simulink model "neurogrip_c0_closed_loop"  (R2026a)
settings: Solver=FixedStepDiscrete  StopTime=0.4  FixedStep=0.02
model workspace (MAT data in the model file):
  c0Mpc = mpc
  c0Mpc.Ts = 0.02
  c0Mpc.PredictionHorizon = 30
  c0Mpc.ControlHorizon = 30
  c0Mpc.Model.Plant = ss
  c0Mpc.Model.Plant.InputName_ = ["steering_angle_rad"; "d_kappa_rad_s"]
  c0Mpc.Model.Plant.InputGroup_.Manipulated = 1
  c0Mpc.Model.Plant.InputGroup_.Measured = 2
  c0Mpc.Model.Plant.OutputName_ = ["e_y_m"; "e_psi_rad"; "v_y_mps"; "yaw_rate_rps"]
  c0Mpc.Model.Plant.OutputGroup_.Measured = [1 2 3 4]
  c0Mpc.Model.Plant.IOSize_ = [4 2]
  c0Mpc.Model.Plant.Data_ = ltipack.ssdata
  c0Mpc.Model.Plant.Data_.a = [1  0.09  0.02  0; 0  1  0  0.02; 0  0  0.463654239616  -0.0414393740331; 0  0  0  0.457235651577]
  c0Mpc.Model.Plant.Data_.c = [1  0  0  0; 0  1  0  0; 0  0  1  0; 0  0  0  1]
  c0Mpc.Model.Plant.Data_.dx0 = [0; 0; 0; 0]
  c0Mpc.Model.Plant.Data_.x0 = [0; 0; 0; 0]
  c0Mpc.Model.Plant.Data_.b = [0  0; 0  -0.02; 1.14394485122  0; 1.59636573066  0]
  c0Mpc.Model.Plant.Data_.d = [0  0; 0  0; 0  0; 0  0]
  c0Mpc.Model.Plant.Data_.u0 = [0; 0]
  c0Mpc.Model.Plant.Data_.y0 = [0; 0; 0; 0]
  c0Mpc.Model.Plant.Data_.Delay.Input = [0; 0]
  c0Mpc.Model.Plant.Data_.Delay.Output = [0; 0; 0; 0]
  c0Mpc.Model.Plant.Data_.Delay.Internal = []
  c0Mpc.Model.Plant.Data_.Ts = 0.02
  c0Mpc.Model.Disturbance = []
  c0Mpc.Model.Noise = []
  c0Mpc.Model.Nominal.X = [0; 0; 0; 0]
  c0Mpc.Model.Nominal.DX = [0; 0; 0; 0]
  c0Mpc.Model.Nominal.U = [0; 0]
  c0Mpc.Model.Nominal.Y = [0; 0; 0; 0]
  c0Mpc.ManipulatedVariables.Min = -0.37
  c0Mpc.ManipulatedVariables.Max = 0.37
  c0Mpc.ManipulatedVariables.MinECR = 0
  c0Mpc.ManipulatedVariables.MaxECR = 0
  c0Mpc.ManipulatedVariables.RateMin = -0.05
  c0Mpc.ManipulatedVariables.RateMax = 0.05
  c0Mpc.ManipulatedVariables.RateMinECR = 0
  c0Mpc.ManipulatedVariables.RateMaxECR = 0
  c0Mpc.ManipulatedVariables.Target = 'nominal'
  c0Mpc.ManipulatedVariables.Name = 'steering_angle_rad'
  c0Mpc.ManipulatedVariables.Units = ''
  c0Mpc.ManipulatedVariables.ScaleFactor = 1
  c0Mpc.ManipulatedVariables.Type = 'continuous'
  c0Mpc.OutputVariables(1).Min = -1.5
  c0Mpc.OutputVariables(1).Max = 1.5
  c0Mpc.OutputVariables(1).MinECR = 1
  c0Mpc.OutputVariables(1).MaxECR = 1
  c0Mpc.OutputVariables(1).Name = 'e_y_m'
  c0Mpc.OutputVariables(1).Units = ''
  c0Mpc.OutputVariables(1).ScaleFactor = 1
  c0Mpc.OutputVariables(2).Min = -Inf
  c0Mpc.OutputVariables(2).Max = Inf
  c0Mpc.OutputVariables(2).MinECR = 1
  c0Mpc.OutputVariables(2).MaxECR = 1
  c0Mpc.OutputVariables(2).Name = 'e_psi_rad'
  c0Mpc.OutputVariables(2).Units = ''
  c0Mpc.OutputVariables(2).ScaleFactor = 1
  c0Mpc.OutputVariables(3).Min = -Inf
  c0Mpc.OutputVariables(3).Max = Inf
  c0Mpc.OutputVariables(3).MinECR = 1
  c0Mpc.OutputVariables(3).MaxECR = 1
  c0Mpc.OutputVariables(3).Name = 'v_y_mps'
  c0Mpc.OutputVariables(3).Units = ''
  c0Mpc.OutputVariables(3).ScaleFactor = 1
  c0Mpc.OutputVariables(4).Min = -Inf
  c0Mpc.OutputVariables(4).Max = Inf
  c0Mpc.OutputVariables(4).MinECR = 1
  c0Mpc.OutputVariables(4).MaxECR = 1
  c0Mpc.OutputVariables(4).Name = 'yaw_rate_rps'
  c0Mpc.OutputVariables(4).Units = ''
  c0Mpc.OutputVariables(4).ScaleFactor = 1
  c0Mpc.DisturbanceVariables.Name = 'd_kappa_rad_s'
  c0Mpc.DisturbanceVariables.Units = ''
  c0Mpc.DisturbanceVariables.ScaleFactor = 1
  c0Mpc.Weights.ManipulatedVariables = 20
  c0Mpc.Weights.ManipulatedVariablesRate = 5
  c0Mpc.Weights.OutputVariables = [40 60 5 10]
  c0Mpc.Weights.ECR = 100000
  c0Mpc.Optimizer.OptimizationType = 'QP'
  c0Mpc.Optimizer.Solver = 'active-set'
  c0Mpc.Optimizer.SolverOptions = mpc.solver.options.qp.ActiveSet
  c0Mpc.Optimizer.SolverOptions.SolverName = 'ActiveSet'
  c0Mpc.Optimizer.MinOutputECR = 0
  c0Mpc.Optimizer.UseSuboptimalSolution = 0
  c0Mpc.Optimizer.CustomSolver = 0
  c0Mpc.Optimizer.CustomSolverCodeGen = 0
  c0Mpc.History = [2026 10 3 11 47 54.765249]
  c0Mpc.MPCData = mpcdata
  c0Mpc.MPCData.IsDirty = 1
  c0Mpc.MPCData.Ts = 0.02
  c0Mpc.MPCData.p = 30
  c0Mpc.MPCData.m = 30
  c0Mpc.MPCData.UseActiveSetSolver = 1
  c0Mpc.MPCData.UseSuboptimalSolution = 0
  c0Mpc.MPCData.CustomSolver = 0
  c0Mpc.MPCData.CustomSolverCodeGen = 0
  c0Mpc.MPCData.IsCustomEstimation = 0
  c0Mpc.MPCData.Uscale = [1; 1]
  c0Mpc.MPCData.Yscale = [1; 1; 1; 1]
  c0Mpc.MPCData.mvindex = 1
  c0Mpc.MPCData.mdindex = 2
  c0Mpc.MPCData.myindex = [1; 2; 3; 4]
  c0Mpc.MPCData.ASOptions.MaxIterations = 120
  c0Mpc.MPCData.ASOptions.ConstraintTolerance = 1e-06
  c0Mpc.MPCData.ASOptions.UseWarmStart = 1
  c0Mpc.MPCData.IPOptions.MaxIterations = 50
  c0Mpc.MPCData.IPOptions.ConstraintTolerance = 1e-06
  c0Mpc.MPCData.IPOptions.OptimalityTolerance = 1e-06
  c0Mpc.MPCData.IPOptions.ComplementarityTolerance = 1e-08
  c0Mpc.MPCData.IPOptions.StepTolerance = 1e-08
  c0Mpc.MPCData.ADOptions.AbsoluteTolerance = 0.001
  c0Mpc.MPCData.ADOptions.RelativeTolerance = 0.001
  c0Mpc.MPCData.ADOptions.MaxIterations = 1000
  c0Mpc.MPCData.ADOptions.RelaxationParameter = 1.6
  c0Mpc.MPCData.ADOptions.PenaltyParameter = 0.1
  c0Mpc.MPCData.ADOptions.StepSize = 1e-06
  c0Mpc.MPCData.ADOptions.PrimalInfeasibilityTolerance = 0.0001
  c0Mpc.MPCData.ADOptions.DualInfeasibilityTolerance = 0.0001
  c0Mpc.MPCData.ADOptions.EnablePolish = 0
  c0Mpc.MPCData.ADOptions.PolishRegularization = 1e-06
  c0Mpc.MPCData.ADOptions.PolishTolerance = 1e-08
  c0Mpc.MPCData.ADOptions.PolishMaxIterations = 3
  c0Mpc.MPCData.MIQPOptions.MaxIterations = 1000
  c0Mpc.MPCData.MIQPOptions.ConstraintTolerance = 1e-06
  c0Mpc.MPCData.MIQPOptions.UseWarmStart = 0
  c0Mpc.MPCData.MIQPOptions.DiscreteConstraintTolerance = 1e-06
  c0Mpc.MPCData.MIQPOptions.RoundingAtRootNode = 1
  c0Mpc.MPCData.MIQPOptions.MaxPendingNodes = 1000
  c0Mpc.IsEmpty = 0
  c0Mpc.OldOVIntegrator = {[]; []; []; []}
  c0Mpc.Version = '26.1'
libraries: mpclib x1
settings Model: Creator=pavel  LastModifiedBy=pavel

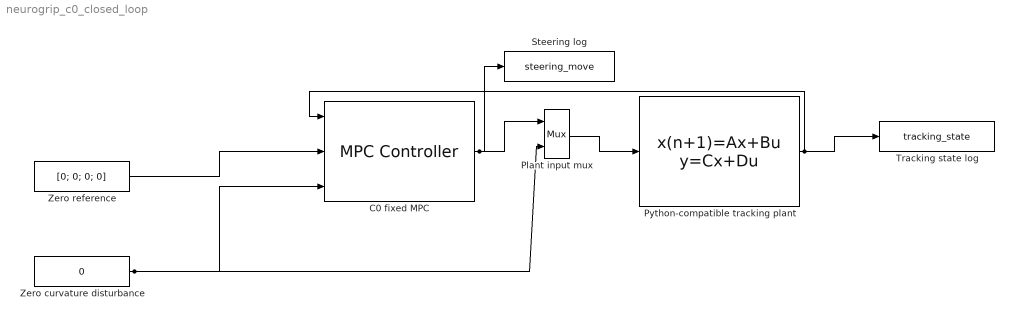
== system neurogrip_c0_closed_loop ==
  C0 fixed MPC : mpclib/MPC Controller  SCDEnableBlockLinearizationSpecification=on  mpcobj=c0Mpc  is_multiple=0  enable_value=0  return_u0=off  updateMPCinCallerWorkspace=on  md_inport=on  mv_inport=off  uref_inport=off  return_cost=off  return_mvseq=off  return_qpstatus=off  return_xseq=off  return_state=off  return_ovseq=off  state_inport=off  umin_inport=off  umax_inport=off  ymin_inport=off  ymax_inport=off  cc_inport=off  ywt_inport=off  uwt_inport=off  duwt_inport=off  rhoeps_inport=off  pm_inport=off  MaximumP=10  HorizonChoice=FixedHorizon  n_ts=1  n_p=10  n_mv=1  n_md=1  n_ud=0  n_mo=1  n_uo=0  BlockDataType=double  SampleTimeInherited=off  switch_inport=off
  Plant input mux : Mux  Inputs=2
  Python-compatible tracking plant : DiscreteStateSpace  A=[1 0.089999999999999997 0.02 0;0 1 0 0.02;0 0 0.46365423961556773 -0.041439374033090781;0 0 0 0.4572356515766039]  B=[0 0;0 -0.02;1.1439448512165971 0;1.5963657306570473 0]  C=eye(4)  D=zeros(4, 2)  InitialCondition=[0.20; 0.05; 0.00; 0.00]  SampleTime=0.02
  Steering log : ToWorkspace  VariableName=steering_move  SaveFormat=Structure With Time  SampleTime=-1
  Tracking state log : ToWorkspace  VariableName=tracking_state  SaveFormat=Structure With Time  SampleTime=-1
  Zero curvature disturbance : Constant  Value=0
  Zero reference : Constant  Value=[0; 0; 0; 0]
  wires:
  Zero reference/1 -> C0 fixed MPC/2
  Zero curvature disturbance/1 -> C0 fixed MPC/3, Plant input mux/2
  C0 fixed MPC/1 -> Plant input mux/1, Steering log/1
  Plant input mux/1 -> Python-compatible tracking plant/1
  Python-compatible tracking plant/1 -> C0 fixed MPC/1, Tracking state log/1
